simulink model "untitled"  (R2018a)
settings: Solver=VariableStepAuto  StartTime=0.0  StopTime=24  RelTol=1e-3
model workspace (MAT data in the model file):
  M_heater_air = Simulink.Parameter
  M_heater_air.Value = 3600
  M_heater_air.DataType = 'auto'
  M_heater_air.Dimensions = [1 1]
  R_equivalent = Simulink.Parameter
  R_equivalent.Value = 4.329e-07
  R_equivalent.DataType = 'auto'
  R_equivalent.Dimensions = [1 1]
  T_heater = Simulink.Parameter
  T_heater.Value = 50
  T_heater.DataType = 'auto'
  T_heater.Dimensions = [1 1]
  Troom_IC = Simulink.Parameter
  Troom_IC.Value = 20
  Troom_IC.DataType = 'auto'
  Troom_IC.Dimensions = [1 1]
  c_air = Simulink.Parameter
  c_air.Value = 1005.4
  c_air.DataType = 'auto'
  c_air.Dimensions = [1 1]
  m_room_air = Simulink.Parameter
  m_room_air.Value = 1470
  m_room_air.DataType = 'auto'
  m_room_air.Dimensions = [1 1]
settings Model: Creator=SH1906014  LastModifiedBy=SH1906014

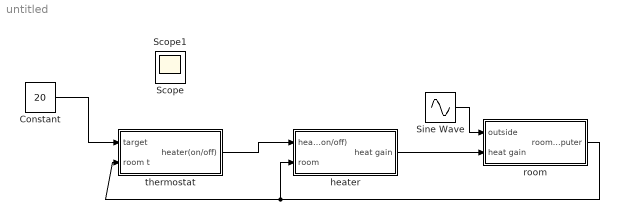
== system untitled ==
  Constant : Constant  Value=20
  Sine Wave : Sin  Amplitude=5  Bias=19  Frequency=2*pi/24  Phase=180  SampleTime=0
  heater : Subsystem
  room : Subsystem
  thermostat : Subsystem
  Scope : Scope
  Scope1 : Scope
  wires:
  heater/1(heat gain) -> room/2(heat gain)
  room/1(room temputer) -> heater/2(room), thermostat/2("room t ")
  thermostat/1(heater(on/off)) -> heater/1(heater(on/off))
  Constant/1 -> thermostat/1(target)
  Sine Wave/1 -> room/1(outside)

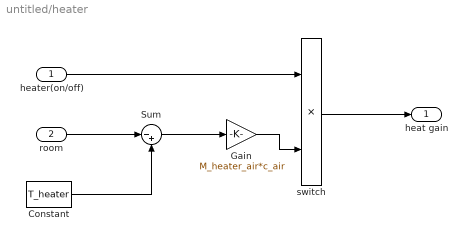
== system untitled/heater ==
  heater(on/off) : Inport
  room : Inport  Port=2
  Constant : Constant  Value=T_heater
  Gain : Gain  Gain=M_heater_air*c_air
  Sum : Sum  Inputs=|-+
  switch : Product
  heat gain : Outport
  wires:
  room/1 -> Sum/1
  Constant/1 -> Sum/2
  Sum/1 -> Gain/1
  heater(on/off)/1 -> switch/1
  switch/1 -> heat gain/1
  Gain/1 -> switch/2

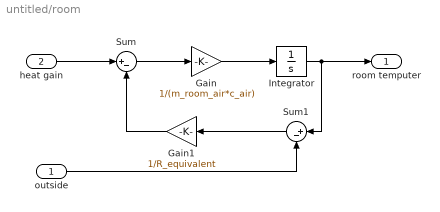
== system untitled/room ==
  outside : Inport
  heat gain : Inport  Port=2
  Gain : Gain  Gain=1/(m_room_air*c_air)
  Gain1 : Gain  Gain=1/R_equivalent
  Integrator : Integrator  InitialCondition=Troom_IC
  Sum : Sum  Inputs=|+-
  Sum1 : Sum  Inputs=|+-
  room temputer : Outport
  wires:
  heat gain/1 -> Sum/1
  Sum/1 -> Gain/1
  Gain/1 -> Integrator/1
  Integrator/1 -> Sum1/1, room temputer/1
  outside/1 -> Sum1/2
  Sum1/1 -> Gain1/1
  Gain1/1 -> Sum/2

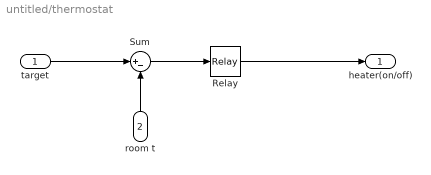
== system untitled/thermostat ==
  target : Inport
  "room t " : Inport  Port=2
  Relay : Relay  OnSwitchValue=2  OffSwitchValue=-2
  Sum : Sum  Inputs=|+-
  heater(on/off) : Outport
  wires:
  target/1 -> Sum/1
  "room t "/1 -> Sum/2
  Sum/1 -> Relay/1
  Relay/1 -> heater(on/off)/1
